simulink library "INT_EngReq_InjLimCalc"  (R2016b)
settings: Solver=VariableStepAuto  StartTime=0.0  StopTime=10.0  RelTol=1e-3
settings Model: Creator=Administrator  LastModifiedBy=Administrator

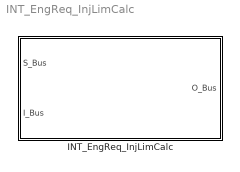
== system INT_EngReq_InjLimCalc ==
  INT_EngReq_InjLimCalc : Subsystem

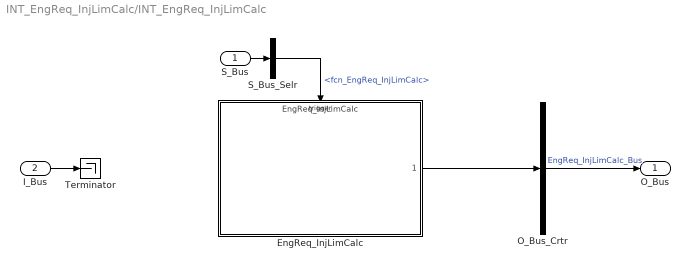
== system INT_EngReq_InjLimCalc/INT_EngReq_InjLimCalc ==
  S_Bus : Inport
  I_Bus : Inport  Port=2
  EngReq_InjLimCalc : ModelReference  ModelNameDialog=EngReq_InjLimCalc  SimulationMode=Normal  ModelReferenceVersion=1.4  TriggerPortName=function  TriggerPortTriggerType=function-call  TriggerPortStatesWhenEnabling=held
  O_Bus_Crtr : BusCreator  Inputs=1
  S_Bus_Selr : BusSelector  OutputSignals=fcn_EngReq_InjLimCalc
  Terminator : Terminator
  O_Bus : Outport
  wires:
  S_Bus_Selr/1 -> EngReq_InjLimCalc/Trigger  "<fcn_EngReq_InjLimCalc>"
  S_Bus/1 -> S_Bus_Selr/1
  I_Bus/1 -> Terminator/1
  O_Bus_Crtr/1 -> O_Bus/1  "EngReq_InjLimCalc_Bus"
  EngReq_InjLimCalc/1 -> O_Bus_Crtr/1
